simulink model "IdleSpeedController"  (R2022a)
settings: Solver=FixedStepAuto  StartTime=0.0  StopTime=10.0  FixedStep=0.01  RelTol=1e-3  EnableMultiTasking=on
InitFcn:
  | IdleSpeedSimParameters
values from neighbouring files (symbols this model uses):
  k = lqr(X,Y,Q,R)    [LQR_Gains.m]
settings Model: Creator=burl  LastModifiedBy=prajw
settings SolverCC: AlgebraicLoopSolver=TrustRegion
settings DataIOCC: ReturnWorkspaceOutputs=off
settings OptimizationCC: LifeSpan=inf
settings DebuggingCC: UnconnectedInputMsg=warning  UnconnectedOutputMsg=warning  UnconnectedLineMsg=warning  SFUnexpectedBacktrackingDiag=warning  SFNoUnconditionalDefaultTransitionDiag=warning  SFMachineParentedDataDiag=warning  ArithmeticOperatorsInVariantConditions=warning
settings SFSimCC: SimUseLocalCustomCode=off  CustomCodeUndefinedFunction=UseInterfaceOnly
settings RTWCC: RTWUseLocalCustomCode=off
settings CodeAppCC: StateflowObjectComments=on
settings GRTTargetCC: TargetLangStandard=C89/C90 (ANSI)
settings ConfigComp: CovMetricSettings=dw  CovSaveCumulativeToWorkspaceVar=on  CovSaveSingleToWorkspaceVar=on  CovExternalEMLEnable=off

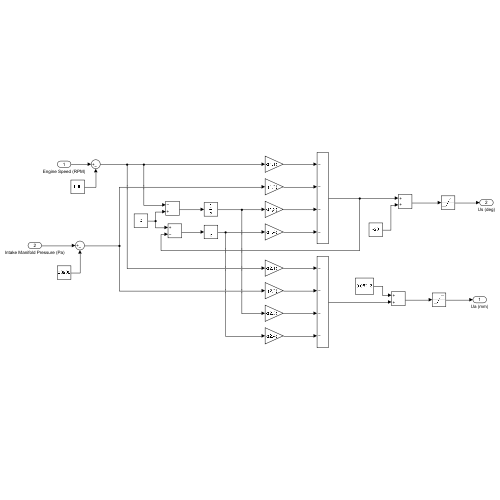
[thumbnail: Simulink's stored preview of the top-level diagram]
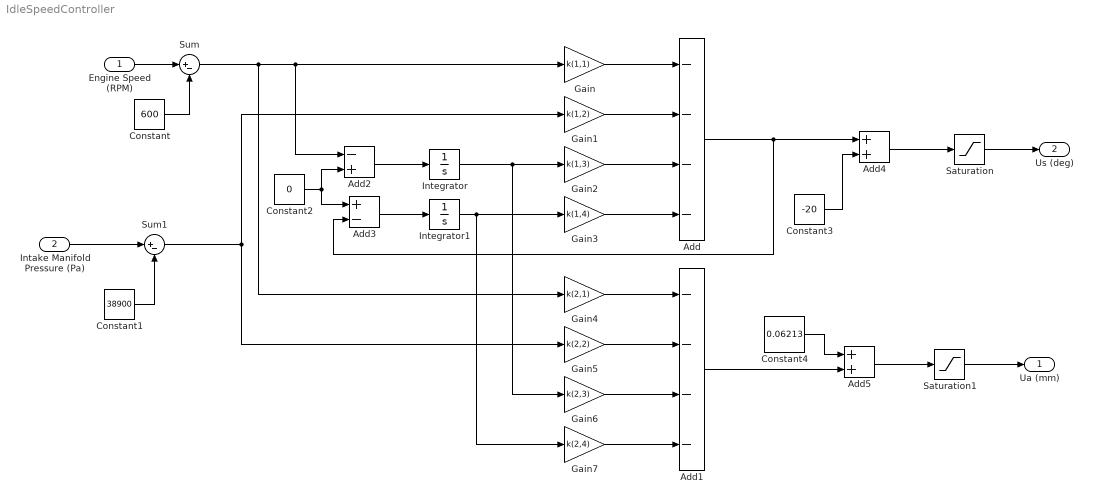
== system IdleSpeedController ==
  Engine Speed (RPM) : Inport
  Intake Manifold Pressure (Pa) : Inport  Port=2
  Add : Sum  Inputs=----
  Add1 : Sum  Inputs=----
  Add2 : Sum  Inputs=-+
  Add3 : Sum  Inputs=+-
  Add4 : Sum
  Add5 : Sum
  Constant : Constant  Value=600
  Constant1 : Constant  Value=38900
  Constant2 : Constant  Value=0
  Constant3 : Constant  Value=-20
  Constant4 : Constant  Value=0.06213
  Gain : Gain  Gain=k(1,1)
  Gain1 : Gain  Gain=k(1,2)
  Gain2 : Gain  Gain=k(1,3)
  Gain3 : Gain  Gain=k(1,4)
  Gain4 : Gain  Gain=k(2,1)
  Gain5 : Gain  Gain=k(2,2)
  Gain6 : Gain  Gain=k(2,3)
  Gain7 : Gain  Gain=k(2,4)
  Integrator : Integrator
  Integrator1 : Integrator
  Saturation : Saturate  UpperLimit=0  LowerLimit=-40
  Saturation1 : Saturate  UpperLimit=0.12  LowerLimit=0
  Sum : Sum  Inputs=|+-
  Sum1 : Sum  Inputs=|+-
  Ua (mm) : Outport  VectorParamsAs1DForOutWhenUnconnected=off
  Us (deg) : Outport  Port=2  VectorParamsAs1DForOutWhenUnconnected=off
  wires:
  Engine Speed (RPM)/1 -> Sum/1
  Constant/1 -> Sum/2
  Sum/1 -> Gain4/1, Add2/1, Gain/1
  Gain/1 -> Add/1
  Gain1/1 -> Add/2
  Gain2/1 -> Add/3
  Gain3/1 -> Add/4
  Gain4/1 -> Add1/1
  Gain5/1 -> Add1/2
  Gain6/1 -> Add1/3
  Gain7/1 -> Add1/4
  Constant2/1 -> Add3/1, Add2/2
  Add2/1 -> Integrator/1
  Add3/1 -> Integrator1/1
  Intake Manifold Pressure (Pa)/1 -> Sum1/1
  Constant1/1 -> Sum1/2
  Sum1/1 -> Gain5/1, Gain1/1
  Integrator/1 -> Gain6/1, Gain2/1
  Integrator1/1 -> Gain7/1, Gain3/1
  Add/1 -> Add3/2, Add4/1
  Constant3/1 -> Add4/2
  Add4/1 -> Saturation/1
  Add1/1 -> Add5/2
  Constant4/1 -> Add5/1
  Add5/1 -> Saturation1/1
  Saturation1/1 -> Ua (mm)/1
  Saturation/1 -> Us (deg)/1
